simulink model "testLtvMpc"  (R2019b)
settings: Solver=VariableStepAuto  StartTime=0.0  StopTime=10  RelTol=1e-3
undefined symbols (not defined in the file or in its folder): A, Au, Ax, B, b, fu, fx, Q, R, T, ulb, uub, x0
settings Model: Creator=louis  LastModifiedBy=louis

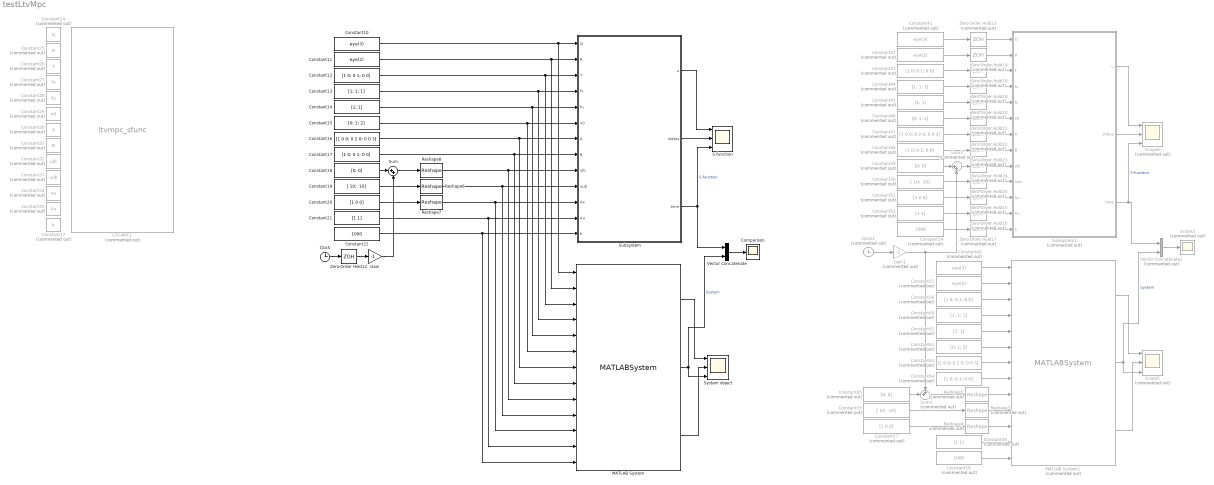
== system testLtvMpc ==
  Clock : Clock
  Clock1 : Clock  Commented=on
  Comparison : Scope
  Constant10 : Constant  Value=eye(3)  SampleTime=0.5
  Constant11 : Constant  Value=eye(2)  SampleTime=0.5
  Constant12 : Constant  Value=[1 0; 0 1; 0 0]  SampleTime=0.5
  Constant13 : Constant  Value=[1; 1; 1]  SampleTime=0.5
  Constant14 : Constant  Value=[1; 1]  SampleTime=0.5
  Constant15 : Constant  Value=[0; 1; 2]  SampleTime=0.5
  Constant16 : Constant  Value=[1 0 0; 0 2 0; 0 0 3]  SampleTime=0.5
  Constant17 : Constant  Value=[1 0; 0 1; 0 0]  SampleTime=0.5
  Constant18 : Constant  Value=[0; 0]  SampleTime=0.5
  Constant19 : Constant  Value="[ 10;  10]"  SampleTime=0.5
  Constant20 : Constant  Value=[1 0 0]  SampleTime=0.5
  Constant21 : Constant  Value=[1 1]  SampleTime=0.5
  Constant22 : Constant  Value=1000  SampleTime=0.5
  Constant24 : Constant  Commented=on  Value=Q
  Constant25 : Constant  Commented=on  Value=R
  Constant26 : Constant  Commented=on  Value=T
  Constant27 : Constant  Commented=on  Value=fx
  Constant28 : Constant  Commented=on  Value=fu
  Constant29 : Constant  Commented=on  Value=x0
  Constant30 : Constant  Commented=on  Value=A
  Constant31 : Constant  Commented=on  Value=B
  Constant32 : Constant  Commented=on  Value=ulb
  Constant33 : Constant  Commented=on  Value=uub
  Constant34 : Constant  Commented=on  Value=Ax
  Constant35 : Constant  Commented=on  Value=Au
  Constant37 : Constant  Commented=on  Value=b
  Constant40 : Constant  Commented=on  Value=eye(3)
  Constant41 : Constant  Commented=on  Value=eye(3)
  Constant42 : Constant  Commented=on  Value=eye(2)
  Constant{43,48,56,64} (4 alike) : Constant  Commented=on  Value=[1 0; 0 1; 0 0]
  Constant44 : Constant  Commented=on  Value=[1; 1; 1]
  Constant45 : Constant  Commented=on  Value=[1; 1]
  Constant46 : Constant  Commented=on  Value=[0; 1; 2]
  Constant47 : Constant  Commented=on  Value=[1 0 0; 0 2 0; 0 0 3]
  Constant49 : Constant  Commented=on  Value=[0; 0]
  Constant50 : Constant  Commented=on  Value="[ 10;  10]"
  Constant51 : Constant  Commented=on  Value=eye(2)
  Constant52 : Constant  Commented=on  Value=[1 0 0]
  Constant53 : Constant  Commented=on  Value=[1 1]
  Constant54 : Constant  Commented=on  Value=1000
  Constant55 : Constant  Commented=on  Value="[ 10;  10]"
  Constant57 : Constant  Commented=on  Value=[1 0 0]
  Constant58 : Constant  Commented=on  Value=[1 1]
  Constant59 : Constant  Commented=on  Value=1000
  Constant60 : Constant  Commented=on  Value=[1; 1; 1]
  Constant61 : Constant  Commented=on  Value=[1; 1]
  Constant62 : Constant  Commented=on  Value=[0; 1; 2]
  Constant63 : Constant  Commented=on  Value=[1 0 0; 0 2 0; 0 0 3]
  Constant65 : Constant  Commented=on  Value=[0; 0]
  Gain : Gain  Gain=-1
  Gain1 : Gain  Commented=on  Gain=-1
  LTV-MPC1 : S-Function  Commented=on  FunctionName=ltvmpc_sfunc  Parameters=Np,Nt,Nx,Nu,Nc,Ns,slackIdx,slackWeight,Ts  SFunctionDeploymentMode=off  EnableBusSupport=off  mask(LTV MPC){Np=10, Nt=5, Nx=3, Nu=2, Nc=1, softConstTable={ '1', '[1]', '1000' }, Ts=1.0}
      mask prompts: Np "Prediction horizon"; Nt "Control horizon"; Nx "Number of states"; Nu "Number of inputs"; Nc "Number of constraints"; softConstTable "Soft constraints"; Ts "Sampling time"
      mask help: Linear Time-Varying MPC
      mask init:
      | % Horizons
      | Np = uint8(Np);
      | Nt = uint8(Nt);
      | 
      | % Matrices size
      | Nx = uint8(Nx);
      | Nu = uint8(Nu);
      | Nc = uint8(Nc);
      | 
      | % Soft constraints
      | softConstTableVal = eval(softConstTable);
      | Ns = size(softConstTableVal,1);
      | slackIdx    = cell(Ns,1);
      | slackWeight = cell(Ns,1);
      | for i = 1:Ns
      |     % Index of soft constraints
      |     thisSlackIdx = eval(softConstTableVal{i,2});
      |     thisSlackIdx = uint8(thisSlackIdx);
      |     slackIdx{i} = thisSlackIdx;
      |     % Penalty weight on the slack variable
      |     thisWeight = eval(softConstTableVal{i,3});
      |     slackWeight{i} = abs(thisWeight);
      | end
      | Ns = uint8(Ns);
      mask DialogControl Container4 Prompt: Hyper-parameters
      mask DialogControl Container7 Prompt: Horizons
      mask DialogControl Container11 Prompt: Model size
      mask DialogControl Container8 Prompt: Polytopic constraints
      mask DialogControl addSlackVar Prompt: Add
      mask DialogControl addSlackVar Callback:
      | % Get block mask handle.
      | maskObj = Simulink.Mask.get(gcb);
      | 
      | % Get custom table handle.
      | tableControl = maskObj.getDialogControl('softConstTable');
      | 
      | % Add a row to the table
      | rowIdx = tableControl.getNumberOfRows();
      | tableControl.addRow(num2str(rowIdx+1),'[1]','1000');
      mask DialogControl delSlackVar Prompt: Delete
      mask DialogControl delSlackVar Callback:
      | % Get block mask handle.
      | maskObj = Simulink.Mask.get(gcb);
      | 
      | % Get custom table handle.
      | tableControl = maskObj.getDialogControl('softConstTable');
      | 
      | % Add a row to the table
      | rowIdx = tableControl.getSelectedRows();
      | for i = 1:numel(rowIdx)
      | 	tableControl.removeRow(rowIdx(i));
      | end
      | 
      | % Renumber rows
      | for i = 1:tableControl.getNumberOfRows()
      |     tableControl.setValue([i 1], num2str(i));
      | end
      mask Display: disp('Linear\nTime-Varying\nMPC')
  MATLAB System : MATLABSystem  System=LTVMPC  hasActuatorBounds=on  hasIneqConstraints=on  hasSoftConstraints=off  softConstraintsIndex={ 0 }  softConstraintsWeight=1e6  Ts=0.5  Nt=10  Np=20  Nx=3  Nu=2  hasScaling=off  actuatorScaling=1  slackScaling=1  hasKnownInput=off  Nw=0  showCost=off  showSolveTime=on  showControlSequence=off  showSlackVariable=off
      mask Type: LTVMPC
      mask Display:
      | disp(['Linear Time' char(10) 'Varying' char(10) 'MPC']);
      | port_label('input',1,'Q');
      | port_label('input',2,'R');
      | port_label('input',3,'T');
      | port_label('input',4,'fx');
      | port_label('input',5,'fu');
      | port_label('input',6,'x0');
      | port_label('input',7,'A');
      | port_label('input',8,'B');
      | port_label('input',9,'ulb');
      | port_label('input',10,'uub');
      | port_label('input',11,'Aineqx');
      | port_label('input',12,'Ainequ');
      | port_label('input',13,'bineq');
      | port_label('output',1,'u_opt');
      | port_label('output',2,'time');
      | port_label('output',3,'status');
  MATLAB System1 : MATLABSystem  Commented=on  System=LTVMPC  hasActuatorBounds=on  hasIneqConstraints=on  hasSoftConstraints=off  softConstraintsIndex={ 0 }  softConstraintsWeight=1e6  Ts=0.5  Nt=15  Np=20  Nx=3  Nu=2  hasScaling=off  actuatorScaling=1  slackScaling=1  hasKnownInput=off  Nw=0  showCost=off  showSolveTime=on  showControlSequence=off  showSlackVariable=off
      mask Type: LTVMPC
      mask Display:
      | disp(['Linear Time' char(10) 'Varying' char(10) 'MPC']);
      | port_label('input',1,'Q');
      | port_label('input',2,'R');
      | port_label('input',3,'T');
      | port_label('input',4,'fx');
      | port_label('input',5,'fu');
      | port_label('input',6,'x0');
      | port_label('input',7,'A');
      | port_label('input',8,'B');
      | port_label('input',9,'ulb');
      | port_label('input',10,'uub');
      | port_label('input',11,'Aineqx');
      | port_label('input',12,'Ainequ');
      | port_label('input',13,'bineq');
      | port_label('output',1,'u_opt');
      | port_label('output',2,'time');
      | port_label('output',3,'status');
  Reshape3 : Reshape  Commented=on  OutputDimensionality=Row vector (2-D)
  Reshape4 : Reshape  Commented=on  OutputDimensionality=Row vector (2-D)
  Reshape5 : Reshape  Commented=on  OutputDimensionality=Row vector (2-D)
  Reshape6 : Reshape  OutputDimensionality=Row vector (2-D)
  Reshape7 : Reshape  OutputDimensionality=Row vector (2-D)
  Reshape8 : Reshape  OutputDimensionality=Row vector (2-D)
  S-function : Scope  NumInputPorts=3
  Scope3 : Scope  Commented=on
  Scope4 : Scope  Commented=on  NumInputPorts=3
  Scope5 : Scope  Commented=on  NumInputPorts=3
  Subsystem : Subsystem  Priority=0  mask(LTV MPC){Np=20, Nt=10, Nx=3, Nu=2, Nc=1, softConstTable={ '1', '[1]', '1000' }, inputScalingTable={ '1', '0', '1'; '2', '0', '1' }, Ts=0.5}
      mask prompts: Np "Prediction horizon"; Nt "Control horizon"; Nx "Number of states"; Nu "Number of inputs"; Nc "Number of constraints"; softConstTable "Soft constraints"; inputScalingTable "Input scaling"; Ts "Sampling time"
      mask help: Linear Time-Varying MPC
      mask init:
      | % Horizons
      | Np = uint8(Np);
      | Nt = uint8(Nt);
      | 
      | % Matrices size
      | Nx = uint8(Nx);
      | Nu = uint8(Nu);
      | Nc = uint8(Nc);
      | 
      | % Soft constraints
      | softConstTableVal = eval(softConstTable);
      | Ns = size(softConstTableVal,1);
      | slackIdx    = cell(Ns,1);
      | slackWeight = cell(Ns,1);
      | for i = 1:Ns
      |     % Index of soft constraints
      |     thisSlackIdx = eval(softConstTableVal{i,2});
      |     thisSlackIdx = uint8(thisSlackIdx);
      |     slackIdx{i} = thisSlackIdx;
      |     % Penalty weight on the slack variable
      |     thisWeight = eval(softConstTableVal{i,3});
      |     slackWeight{i} = abs(thisWeight);
      | end
      | Ns = uint8(Ns);
      | 
      | % Scaling factors
      | inputScalingTableVal = eval(inputScalingTable);
      | inputScaling = zeros(Nu,1);
      | for i = 1:Nu
      |     inputScaling(i) = eval(inputScalingTableVal{i,3});
      | end
      mask Callback Nu:
      | % Get block mask handle.
      | maskObj = Simulink.Mask.get(gcb);
      | 
      | % Get custom table handle.
      | tableControl = maskObj.getDialogControl('inputScalingTable');
      | nbRows = tableControl.getNumberOfRows();
      | 
      | % Get number of inputs
      | Nu = eval(get_param(gcb,'Nu'));
      | 
      | % Delete rows if there are too many
      | for i = flip((Nu+1):nbRows)
      |     tableControl.removeRow(i);
      | end
      | 
      | % Add rows if there are not enough
      | for i = (nbRows+1):Nu
      |     tableControl.addRow(num2str(i),'0','1');
      | end
      | 
      | % Renumber the channels
      | for i = 1:tableControl.getNumberOfRows()
      |     tableControl.setValue([i 1], num2str(i));
      | end
      mask DialogControl paramTab Prompt: Hyper-parameters
      mask DialogControl horizonGroup Prompt: Horizons
      mask DialogControl sizeGroup Prompt: Model size
      mask DialogControl constTab Prompt: Polytopic constraints
      mask DialogControl addSlackVar Prompt: Add
      mask DialogControl addSlackVar Callback:
      | % Get block mask handle.
      | maskObj = Simulink.Mask.get(gcb);
      | 
      | % Get custom table handle.
      | tableControl = maskObj.getDialogControl('softConstTable');
      | 
      | % Add a row to the table
      | rowIdx = tableControl.getNumberOfRows();
      | tableControl.addRow(num2str(rowIdx+1),'[1]','1000');
      mask DialogControl delSlackVar Prompt: Delete
      mask DialogControl delSlackVar Callback:
      | % Get block mask handle.
      | maskObj = Simulink.Mask.get(gcb);
      | 
      | % Get custom table handle.
      | tableControl = maskObj.getDialogControl('softConstTable');
      | 
      | % Add a row to the table
      | rowIdx = tableControl.getSelectedRows();
      | for i = 1:numel(rowIdx)
      | 	tableControl.removeRow(rowIdx(i));
      | end
      | 
      | % Renumber rows
      | for i = 1:tableControl.getNumberOfRows()
      |     tableControl.setValue([i 1], num2str(i));
      | end
      mask DialogControl scalingTab Prompt: Scaling
      mask Display: disp('Linear\nTime-Varying\nMPC')
  Subsystem1 : Subsystem  Commented=on  mask(LTV MPC){Np=20, Nt=15, Nx=3, Nu=2, Nc=1, softConstTable={ '1', '[1]', '1000' }, inputScalingTable={ '1', '0', '1'; '2', '0', '1' }, Ts=0.5}
      mask prompts: Np "Prediction horizon"; Nt "Control horizon"; Nx "Number of states"; Nu "Number of inputs"; Nc "Number of constraints"; softConstTable "Soft constraints"; inputScalingTable "Input scaling"; Ts "Sampling time"
      mask help: Linear Time-Varying MPC
      mask init: same as testLtvMpc/LTV-MPC1
      mask Callback Nu:
      | % Get block mask handle.
      | maskObj = Simulink.Mask.get(gcb);
      | 
      | % Get custom table handle.
      | tableControl = maskObj.getDialogControl('inputScalingTable');
      | nbRows = tableControl.getNumberOfRows();
      | 
      | % Get number of inputs
      | Nu = eval(get_param(gcb,'Nu'));
      | 
      | % Delete rows if there are too many
      | for i = flip((Nu+1):nbRows)
      |     tableControl.removeRow(i);
      | end
      | 
      | % Add rows if there are not enough
      | for i = (nbRows+1):Nu
      |     tableControl.addRow(num2str(i),'0','1');
      | end
      | 
      | % Renumber the channels
      | for i = 1:tableControl.getNumberOfRows()
      |     tableControl.setValue([i 1], num2str(i));
      | end
      mask DialogControl paramTab Prompt: Hyper-parameters
      mask DialogControl horizonGroup Prompt: Horizons
      mask DialogControl sizeGroup Prompt: Model size
      mask DialogControl constTab Prompt: Polytopic constraints
      mask DialogControl addSlackVar Prompt: Add
      mask DialogControl addSlackVar Callback:
      | % Get block mask handle.
      | maskObj = Simulink.Mask.get(gcb);
      | 
      | % Get custom table handle.
      | tableControl = maskObj.getDialogControl('softConstTable');
      | 
      | % Add a row to the table
      | rowIdx = tableControl.getNumberOfRows();
      | tableControl.addRow(num2str(rowIdx+1),'[1]','1000');
      mask DialogControl delSlackVar Prompt: Delete
      mask DialogControl delSlackVar Callback:
      | % Get block mask handle.
      | maskObj = Simulink.Mask.get(gcb);
      | 
      | % Get custom table handle.
      | tableControl = maskObj.getDialogControl('softConstTable');
      | 
      | % Add a row to the table
      | rowIdx = tableControl.getSelectedRows();
      | for i = 1:numel(rowIdx)
      | 	tableControl.removeRow(rowIdx(i));
      | end
      | 
      | % Renumber rows
      | for i = 1:tableControl.getNumberOfRows()
      |     tableControl.setValue([i 1], num2str(i));
      | end
      mask DialogControl scalingTab Prompt: Scaling
      mask Display: disp('Linear\nTime-Varying\nMPC')
  Sum : Sum  Inputs=|++
  Sum2 : Sum  Commented=on  Inputs=|++
  Sum3 : Sum  Commented=on  Inputs=++|
  System object : Scope  NumInputPorts=3
  Vector Concatenate : Concatenate
  Vector Concatenate1 : Concatenate  Commented=on
  Zero-Order Hold12 : ZeroOrderHold  SampleTime=0.5
  Zero-Order Hold{13..25} (13 alike) : ZeroOrderHold  Commented=on  SampleTime=0.5
  wires:
  Constant18/1 -> Sum/1
  Subsystem/1(u) -> S-function/1
  Subsystem/2(status) -> S-function/2
  Subsystem/3(time) -> Vector Concatenate/1, S-function/3  "S-function"
  Constant10/1 -> MATLAB System/1, Subsystem/1(Q)
  Constant11/1 -> MATLAB System/2, Subsystem/2(R)
  Constant12/1 -> MATLAB System/3, Subsystem/3(T)
  Constant13/1 -> MATLAB System/4, Subsystem/4(fx)
  Constant14/1 -> MATLAB System/5, Subsystem/5(fu)
  Constant15/1 -> MATLAB System/6, Subsystem/6(x0)
  Constant16/1 -> MATLAB System/7, Subsystem/7(A)
  Constant17/1 -> MATLAB System/8, Subsystem/8(B)
  Constant21/1 -> MATLAB System/12, Subsystem/12(Au)
  Constant22/1 -> MATLAB System/13, Subsystem/13(b)
  MATLAB System/2 -> Vector Concatenate/2, System object/3  "System"
  MATLAB System/1 -> System object/1
  MATLAB System/3 -> System object/2
  Reshape6/1 -> MATLAB System/10, Subsystem/10(uub)
  Reshape7/1 -> MATLAB System/11, Subsystem/11(Ax)
  Vector Concatenate/1 -> Comparison/1
  Sum/1 -> Reshape8/1
  Constant19/1 -> Reshape6/1
  Constant20/1 -> Reshape7/1
  Clock/1 -> Zero-Order Hold12/1
  Gain/1 -> Sum/2
  Reshape8/1 -> MATLAB System/9, Subsystem/9(ulb)
  Vector Concatenate1/1 -> Scope3/1
  Reshape3/1 -> MATLAB System1/10
  Constant55/1 -> Reshape3/1
  Constant57/1 -> Reshape4/1
  Zero-Order Hold18/1 -> Subsystem1/3(T)
  MATLAB System1/1 -> Scope5/1
  Zero-Order Hold14/1 -> Subsystem1/2(R)
  Zero-Order Hold24/1 -> Subsystem1/9(ulb)
  Constant59/1 -> MATLAB System1/13
  Zero-Order Hold20/1 -> Subsystem1/5(fu)
  Constant41/1 -> Zero-Order Hold13/1
  Constant61/1 -> MATLAB System1/5
  MATLAB System1/3 -> Scope5/2
  Constant52/1 -> Zero-Order Hold15/1
  Constant58/1 -> MATLAB System1/12
  Constant42/1 -> Zero-Order Hold14/1
  Reshape5/1 -> MATLAB System1/9
  MATLAB System1/2 -> Vector Concatenate1/2, Scope5/3  "System"
  Constant60/1 -> MATLAB System1/4
  Constant49/1 -> Sum2/1
  Constant45/1 -> Zero-Order Hold20/1
  Constant46/1 -> Zero-Order Hold21/1
  Sum2/1 -> Zero-Order Hold24/1
  Clock1/1 -> Gain1/1
  Constant43/1 -> Zero-Order Hold18/1
  Constant40/1 -> MATLAB System1/1
  Constant56/1 -> MATLAB System1/3
  Reshape4/1 -> MATLAB System1/11
  Constant54/1 -> Zero-Order Hold17/1
  Zero-Order Hold19/1 -> Subsystem1/4(fx)
  Constant44/1 -> Zero-Order Hold19/1
  Zero-Order Hold22/1 -> Subsystem1/7(A)
  Constant53/1 -> Zero-Order Hold16/1
  Zero-Order Hold21/1 -> Subsystem1/6(x0)
  Subsystem1/1(u) -> Scope4/1
  Constant47/1 -> Zero-Order Hold22/1
  Zero-Order Hold23/1 -> Subsystem1/8(B)
  Constant50/1 -> Zero-Order Hold25/1
  Constant48/1 -> Zero-Order Hold23/1
  Subsystem1/2(status) -> Scope4/2
  Subsystem1/3(time) -> Vector Concatenate1/1, Scope4/3  "S-function"
  Constant64/1 -> MATLAB System1/8
  Constant51/1 -> MATLAB System1/2
  Constant63/1 -> MATLAB System1/7
  Constant62/1 -> MATLAB System1/6
  Zero-Order Hold25/1 -> Subsystem1/10(uub)
  Zero-Order Hold15/1 -> Subsystem1/11(Ax)
  Zero-Order Hold13/1 -> Subsystem1/1(Q)
  Zero-Order Hold17/1 -> Subsystem1/13(b)
  Zero-Order Hold16/1 -> Subsystem1/12(Au)
  Gain1/1 -> Sum3/1, Sum2/2
  Sum3/1 -> Reshape5/1
  Constant65/1 -> Sum3/2
  Zero-Order Hold12/1 -> Gain/1

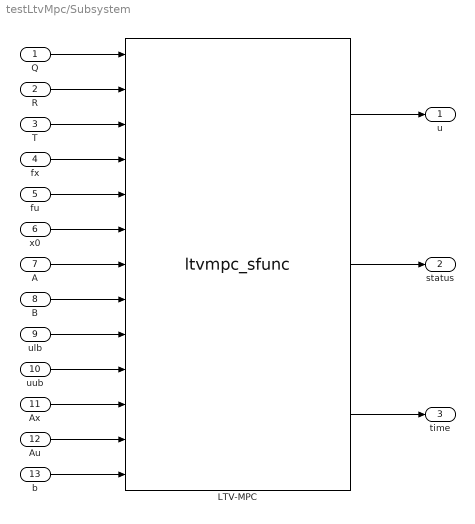
== system testLtvMpc/Subsystem ==
  Q : Inport
  R : Inport  Port=2
  T : Inport  Port=3
  fx : Inport  Port=4
  fu : Inport  Port=5
  x0 : Inport  Port=6
  A : Inport  Port=7
  B : Inport  Port=8
  ulb : Inport  Port=9
  uub : Inport  Port=10
  Ax : Inport  Port=11
  Au : Inport  Port=12
  b : Inport  Port=13
  LTV-MPC : S-Function  FunctionName=ltvmpc_sfunc  Parameters=Np,Nt,Nx,Nu,Nc,Ns,slackIdx,slackWeight,inputScaling,Ts  SFunctionDeploymentMode=off  EnableBusSupport=off
  u : Outport
  status : Outport  Port=2
  time : Outport  Port=3
  wires:
  ulb/1 -> LTV-MPC/9
  LTV-MPC/1 -> u/1
  LTV-MPC/2 -> status/1
  uub/1 -> LTV-MPC/10
  B/1 -> LTV-MPC/8
  fx/1 -> LTV-MPC/4
  Ax/1 -> LTV-MPC/11
  x0/1 -> LTV-MPC/6
  Q/1 -> LTV-MPC/1
  A/1 -> LTV-MPC/7
  R/1 -> LTV-MPC/2
  Au/1 -> LTV-MPC/12
  b/1 -> LTV-MPC/13
  T/1 -> LTV-MPC/3
  fu/1 -> LTV-MPC/5
  LTV-MPC/3 -> time/1

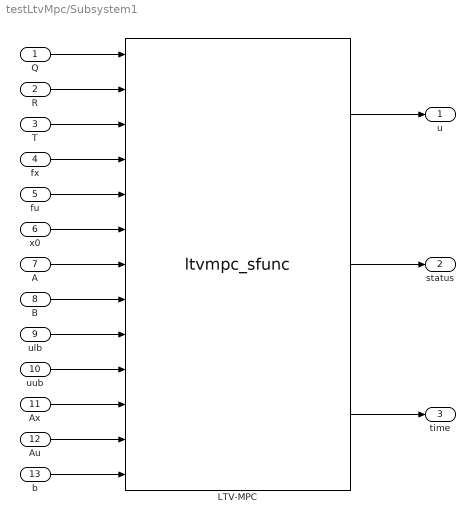
== system testLtvMpc/Subsystem1 ==
  Q : Inport
  R : Inport  Port=2
  T : Inport  Port=3
  fx : Inport  Port=4
  fu : Inport  Port=5
  x0 : Inport  Port=6
  A : Inport  Port=7
  B : Inport  Port=8
  ulb : Inport  Port=9
  uub : Inport  Port=10
  Ax : Inport  Port=11
  Au : Inport  Port=12
  b : Inport  Port=13
  LTV-MPC : S-Function  FunctionName=ltvmpc_sfunc  Parameters=Np,Nt,Nx,Nu,Nc,Ns,slackIdx,slackWeight,Ts  SFunctionDeploymentMode=off  EnableBusSupport=off
  u : Outport
  status : Outport  Port=2
  time : Outport  Port=3
  wires:
  ulb/1 -> LTV-MPC/9
  LTV-MPC/1 -> u/1
  LTV-MPC/2 -> status/1
  uub/1 -> LTV-MPC/10
  B/1 -> LTV-MPC/8
  fx/1 -> LTV-MPC/4
  Ax/1 -> LTV-MPC/11
  x0/1 -> LTV-MPC/6
  Q/1 -> LTV-MPC/1
  A/1 -> LTV-MPC/7
  R/1 -> LTV-MPC/2
  Au/1 -> LTV-MPC/12
  b/1 -> LTV-MPC/13
  T/1 -> LTV-MPC/3
  fu/1 -> LTV-MPC/5
  LTV-MPC/3 -> time/1
